simulink model "MRAC_Augmented_Error_Solution_Unknown_control_gain"  (R2023b)
settings: Solver=FixedStepAuto  StartTime=0.0  StopTime=300  FixedStep=1e-3  RelTol=1e-3
values from neighbouring files (symbols this model uses):
  a0 = 6    [value_tuning.m]
  a1 = 7    [value_tuning.m]
  b0 = 6    [value_tuning.m]
  k0 = 3    [value_tuning.m]
  k_M0 = 1    [value_tuning.m]
  k_M1 = 2    [value_tuning.m]
undefined symbols (not defined in the file or in its folder): gamma1, gamma2
settings Model: Creator=nguye  LastModifiedBy=nguye

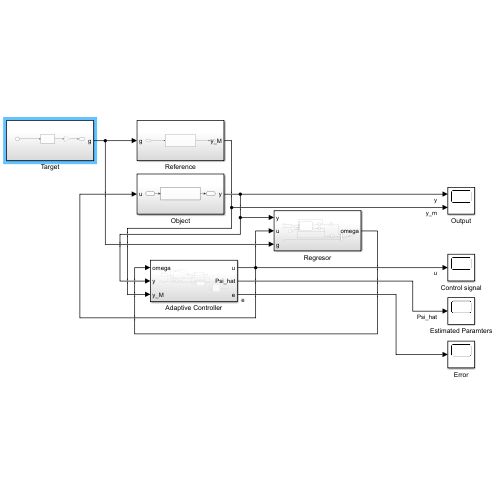
[thumbnail: Simulink's stored preview of the top-level diagram]
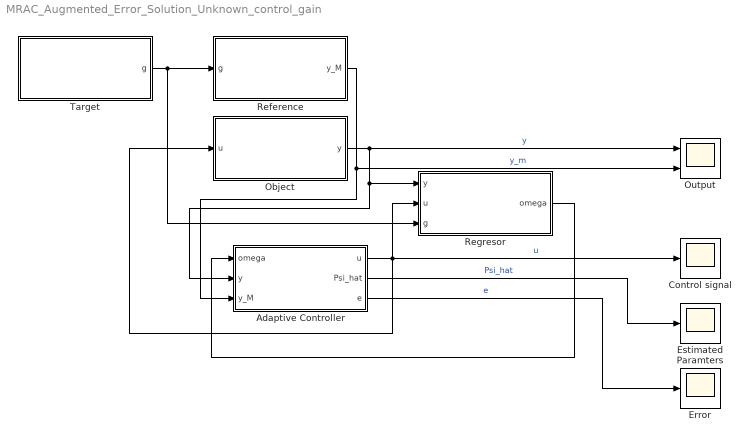
== system MRAC_Augmented_Error_Solution_Unknown_control_gain ==
  Adaptive Controller : Subsystem
  Control signal : Scope
  Error : Scope
  Estimated Paramters : Scope
  Object : Subsystem
  Output : Scope  NumInputPorts=2
  Reference : Subsystem
  Regresor : Subsystem
  Target : Subsystem
  wires:
  Object/1(y) -> Adaptive Controller/2(y), Regresor/1(y), Output/1  "y"
  Adaptive Controller/1(u) -> Regresor/2(u), Control signal/1, Object/1(u)  "u"
  Target/1(g) -> Reference/1(g), Regresor/3(g)
  Regresor/1(omega) -> Adaptive Controller/1(omega)
  Reference/1(y_M) -> Adaptive Controller/3(y_M), Output/2  "y_m"
  Adaptive Controller/2(Psi_hat) -> Estimated Paramters/1  "Psi_hat"
  Adaptive Controller/3(e) -> Error/1  "e"

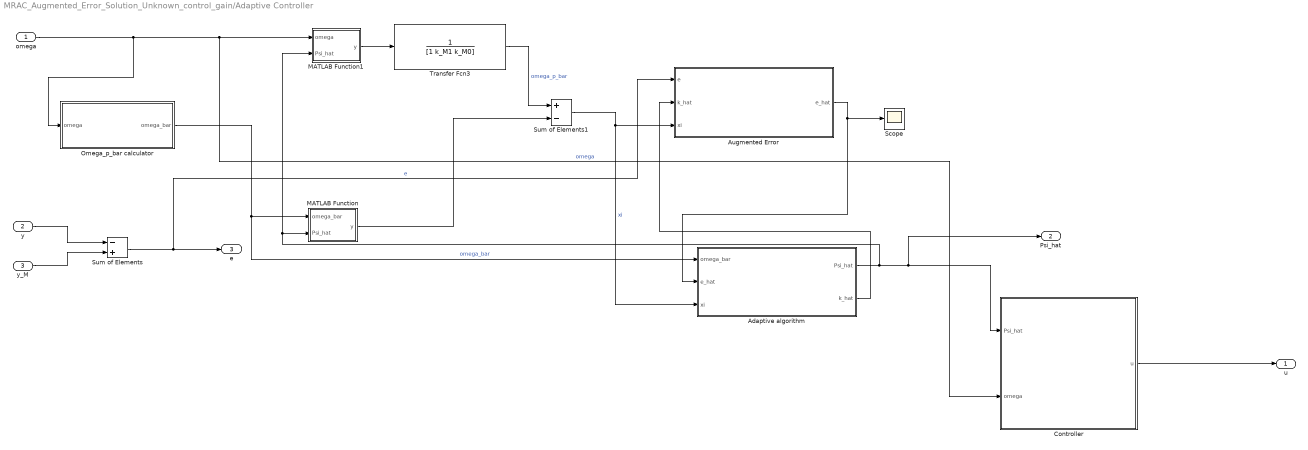
== system MRAC_Augmented_Error_Solution_Unknown_control_gain/Adaptive Controller ==
  omega : Inport
  y : Inport  Port=2
  y_M : Inport  Port=3
  Adaptive algorithm : Subsystem
  Augmented Error : Subsystem
  Controller : MATLAB Function  TreatAsAtomicUnit=on
  MATLAB Function : MATLAB Function  TreatAsAtomicUnit=on
  MATLAB Function1 : MATLAB Function  TreatAsAtomicUnit=on
  Omega_p_bar calculator : Subsystem
  Scope : Scope
  Sum of Elements : Sum  Inputs=-+
  Sum of Elements1 : Sum  Inputs=+-
  Transfer Fcn3 : TransferFcn  Denominator=[1 k_M1 k_M0]
  u : Outport
  Psi_hat : Outport  Port=2
  e : Outport  Port=3
  wires:
  omega/1 -> Controller/2(omega), MATLAB Function1/1(omega), Omega_p_bar calculator/1(omega)  "omega"
  y_M/1 -> Sum of Elements/2
  y/1 -> Sum of Elements/1
  Sum of Elements/1 -> Augmented Error/1(e), e/1  "e"
  Omega_p_bar calculator/1(omega_bar) -> Adaptive algorithm/1(omega_bar), MATLAB Function/1(omega_bar)  "omega_bar"
  Adaptive algorithm/1(Psi_hat) -> MATLAB Function1/2(Psi_hat), MATLAB Function/2(Psi_hat), Controller/1(Psi_hat), Psi_hat/1
  Controller/1(u) -> u/1
  Augmented Error/1(e_hat) -> Adaptive algorithm/2(e_hat), Scope/1
  MATLAB Function1/1(y) -> Transfer Fcn3/1
  MATLAB Function/1(y) -> Sum of Elements1/2
  Transfer Fcn3/1 -> Sum of Elements1/1  "omega_p_bar"
  Sum of Elements1/1 -> Adaptive algorithm/3(xi), Augmented Error/3(xi)  "xi"
  Adaptive algorithm/2(k_hat) -> Augmented Error/2(k_hat)

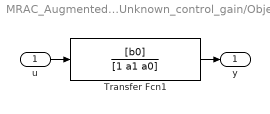
== system MRAC_Augmented_Error_Solution_Unknown_control_gain/Object ==
  u : Inport
  Transfer Fcn1 : TransferFcn  Numerator=[b0]  Denominator=[1 a1 a0]
  y : Outport
  wires:
  u/1 -> Transfer Fcn1/1
  Transfer Fcn1/1 -> y/1

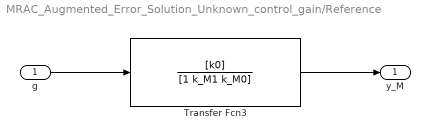
== system MRAC_Augmented_Error_Solution_Unknown_control_gain/Reference ==
  g : Inport
  Transfer Fcn3 : TransferFcn  Numerator=[k0]  Denominator=[1 k_M1 k_M0]
  y_M : Outport
  wires:
  g/1 -> Transfer Fcn3/1
  Transfer Fcn3/1 -> y_M/1

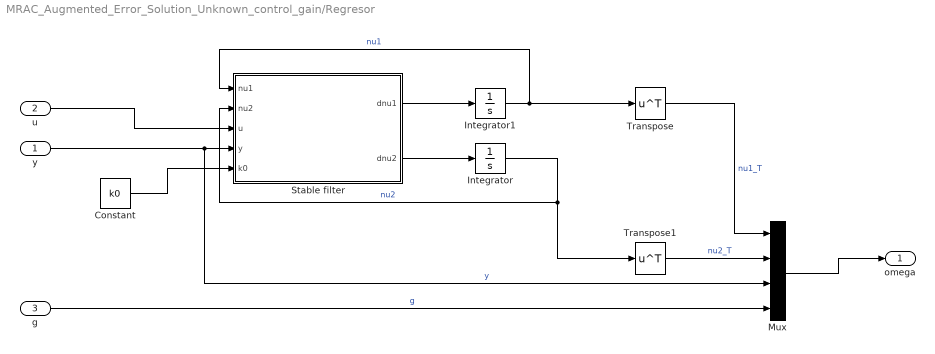
== system MRAC_Augmented_Error_Solution_Unknown_control_gain/Regresor ==
  y : Inport
  u : Inport  Port=2
  g : Inport  Port=3
  Constant : Constant  Value=k0
  Integrator : Integrator
  Integrator1 : Integrator
  Mux : Mux
  Stable filter : MATLAB Function  TreatAsAtomicUnit=on
  Transpose : Math  Operator=transpose
  Transpose1 : Math  Operator=transpose
  omega : Outport
  wires:
  u/1 -> Stable filter/3(u)
  y/1 -> Mux/3, Stable filter/4(y)  "y"
  Stable filter/2(dnu2) -> Integrator/1
  Stable filter/1(dnu1) -> Integrator1/1
  Integrator1/1 -> Stable filter/1(nu1), Transpose/1  "nu1"
  Integrator/1 -> Transpose1/1, Stable filter/2(nu2)  "nu2"
  Mux/1 -> omega/1
  Transpose/1 -> Mux/1  "nu1_T"
  Transpose1/1 -> Mux/2  "nu2_T"
  Constant/1 -> Stable filter/5(k0)
  g/1 -> Mux/4  "g"

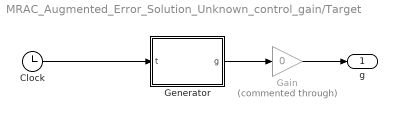
== system MRAC_Augmented_Error_Solution_Unknown_control_gain/Target ==
  Clock : Clock
  Gain : Gain  Commented=through  Gain=0
  Generator : MATLAB Function  TreatAsAtomicUnit=on
  g : Outport
  wires:
  Generator/1(g) -> Gain/1
  Clock/1 -> Generator/1(t)
  Gain/1 -> g/1

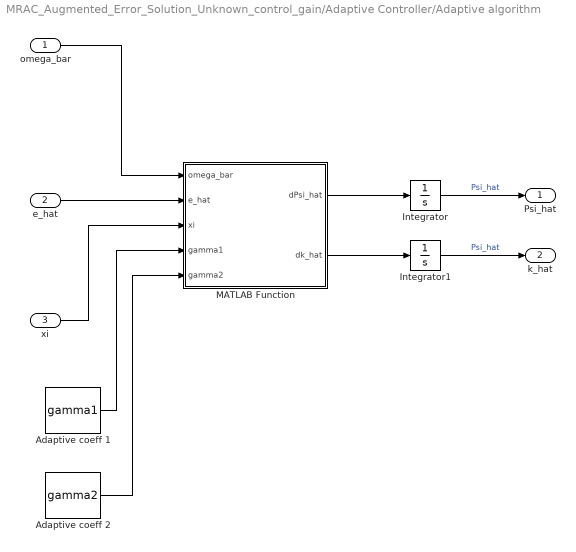
== system MRAC_Augmented_Error_Solution_Unknown_control_gain/Adaptive Controller/Adaptive algorithm ==
  omega_bar : Inport
  e_hat : Inport  Port=2
  xi : Inport  Port=3
  Adaptive coeff 1 : Constant  Value=gamma1
  Adaptive coeff 2 : Constant  Value=gamma2
  Integrator : Integrator
  Integrator1 : Integrator
  MATLAB Function : MATLAB Function  TreatAsAtomicUnit=on
  Psi_hat : Outport
  k_hat : Outport  Port=2
  wires:
  omega_bar/1 -> MATLAB Function/1(omega_bar)
  e_hat/1 -> MATLAB Function/2(e_hat)
  MATLAB Function/1(dPsi_hat) -> Integrator/1
  Integrator/1 -> Psi_hat/1  "Psi_hat"
  Adaptive coeff 1/1 -> MATLAB Function/4(gamma1)
  MATLAB Function/2(dk_hat) -> Integrator1/1
  Integrator1/1 -> k_hat/1  "Psi_hat"
  Adaptive coeff 2/1 -> MATLAB Function/5(gamma2)
  xi/1 -> MATLAB Function/3(xi)

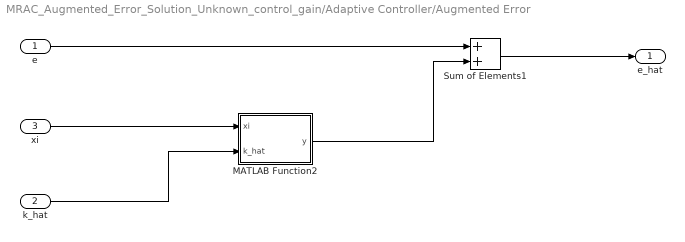
== system MRAC_Augmented_Error_Solution_Unknown_control_gain/Adaptive Controller/Augmented Error ==
  e : Inport
  k_hat : Inport  Port=2
  xi : Inport  Port=3
  MATLAB Function2 : MATLAB Function  TreatAsAtomicUnit=on
  Sum of Elements1 : Sum
  e_hat : Outport
  wires:
  k_hat/1 -> MATLAB Function2/2(k_hat)
  MATLAB Function2/1(y) -> Sum of Elements1/2
  Sum of Elements1/1 -> e_hat/1
  xi/1 -> MATLAB Function2/1(xi)
  e/1 -> Sum of Elements1/1

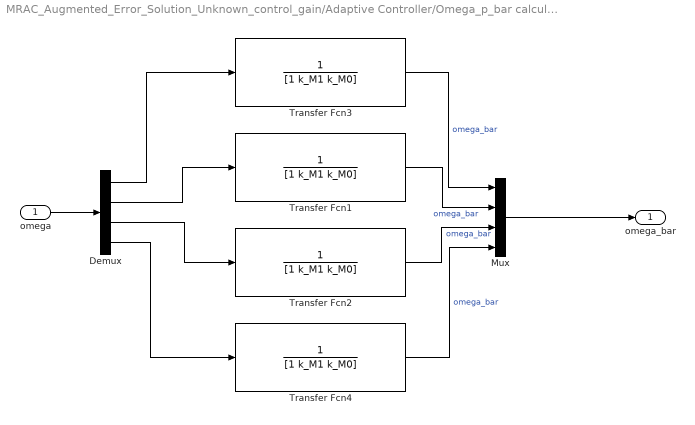
== system MRAC_Augmented_Error_Solution_Unknown_control_gain/Adaptive Controller/Omega_p_bar calculator ==
  omega : Inport
  Demux : Demux
  Mux : Mux
  Transfer Fcn{1..4} (4 alike) : TransferFcn  Denominator=[1 k_M1 k_M0]
  omega_bar : Outport
  wires:
  Demux/1 -> Transfer Fcn3/1
  Demux/2 -> Transfer Fcn1/1
  Demux/3 -> Transfer Fcn2/1
  omega/1 -> Demux/1
  Transfer Fcn1/1 -> Mux/2  "omega_bar"
  Transfer Fcn3/1 -> Mux/1  "omega_bar"
  Transfer Fcn2/1 -> Mux/3  "omega_bar"
  Mux/1 -> omega_bar/1
  Demux/4 -> Transfer Fcn4/1
  Transfer Fcn4/1 -> Mux/4  "omega_bar"

== matlab function MRAC_Augmented_Error_Solution_Unknown_control_gain/Target/Generator ==
  data: t input; g output
function g = fcn(t)

g = 3*sign(sin(0.5*t));

== matlab function MRAC_Augmented_Error_Solution_Unknown_control_gain/Regresor/Stable filter ==
  data: nu1 input; nu2 input; u input; dnu1 output; y input; dnu2 output; k0 input
function [dnu1, dnu2] = fcn(nu1, nu2, u, y, k0)
%
% Stable filters in Lemma (R. V. Monopoli, 1974, direct control parameterization lemma )
%

%
Lambda = -k0;
dnu1 = Lambda*nu1 + u; 
dnu2 = Lambda*nu2 + y;

== matlab function MRAC_Augmented_Error_Solution_Unknown_control_gain/Adaptive Controller/Adaptive algorithm/MATLAB Function ==
  data: omega_bar input; dPsi_hat output; e_hat input; xi input; gamma1 input; gamma2 input; dk_hat output
function [dPsi_hat, dk_hat] = fcn(omega_bar, e_hat, xi, gamma1, gamma2)

dPsi_hat = gamma1 / (1 + omega_bar'*omega_bar) * (omega_bar  .* e_hat);
dk_hat = -gamma2 / (1 + omega_bar'*omega_bar) * (xi .* e_hat);

== matlab function MRAC_Augmented_Error_Solution_Unknown_control_gain/Adaptive Controller/Controller ==
  data: Psi_hat input; u output; omega input
function u = fcn(Psi_hat, omega)

u = Psi_hat'*omega;

== matlab function MRAC_Augmented_Error_Solution_Unknown_control_gain/Adaptive Controller/MATLAB Function ==
  data: omega_bar input; y output; Psi_hat input
function y = fcn(omega_bar, Psi_hat)

y = Psi_hat'*omega_bar;

== matlab function MRAC_Augmented_Error_Solution_Unknown_control_gain/Adaptive Controller/MATLAB Function1 ==
  data: omega input; y output; Psi_hat input
function y = fcn(omega, Psi_hat)

y = Psi_hat'*omega;

== matlab function MRAC_Augmented_Error_Solution_Unknown_control_gain/Adaptive Controller/Augmented Error/MATLAB Function2 ==
  data: xi input; y output; k_hat input
function y = fcn(xi, k_hat)

y = k_hat.*xi;
